simulink model "eval_ekf"  (R2026a)
settings: Solver=VariableStepAuto  StopTime=500
undefined symbols (not defined in the file): ekf_param, perturbed_plant_param, pf_param, r_param, random_seed, u_noise_param
libraries: lib_sensors x6, lib_plant x1
settings Model: SimulationMode=accelerator  Creator=alessandro-nardin  LastModifiedBy=fiore
settings RTWCC: Toolchain=Microsoft Visual C++ 2022 v17.0 | nmake (64-bit Windows)

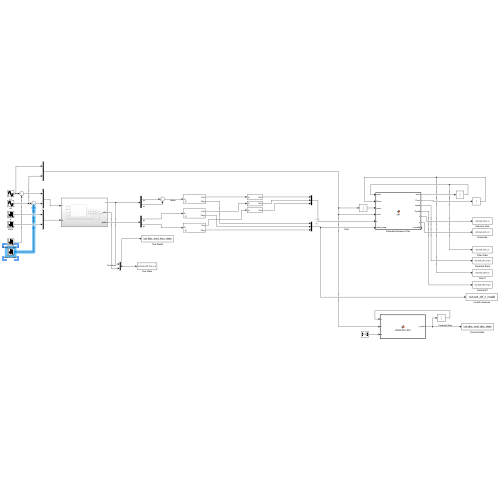
[thumbnail: Simulink's stored preview of the top-level diagram]
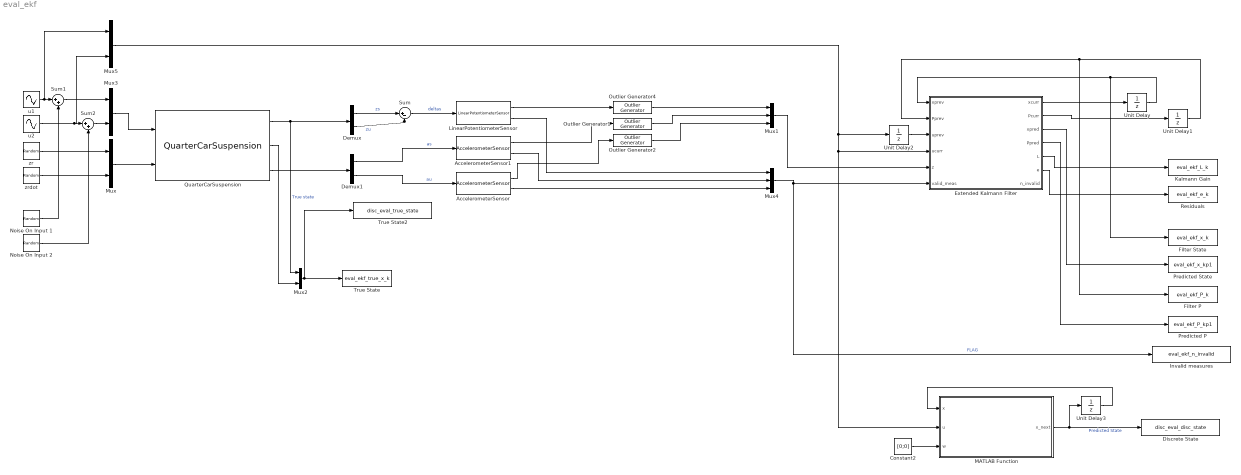
== system eval_ekf ==
  AccelerometerSensor : lib_sensors/AccelerometerSensor  out_sample_t=ekf_param.sample_t
  AccelerometerSensor1 : lib_sensors/AccelerometerSensor  out_sample_t=ekf_param.sample_t
  Constant2 : Constant  Value=[0;0]
  Demux : Demux  Outputs=2
  Demux1 : Demux  Outputs=2
  Discrete State : ToWorkspace  VariableName=disc_eval_disc_state  SaveFormat=Timeseries  SampleTime=ekf_param.sample_t
  Extended Kalmann Filter : MATLAB Function  TreatAsAtomicUnit=on
  Filter P : ToWorkspace  VariableName=eval_ekf_P_k  SaveFormat=Timeseries  SampleTime=1/ekf_param.freq
  Filter State : ToWorkspace  VariableName=eval_ekf_x_k  SaveFormat=Timeseries  SampleTime=1/ekf_param.freq
  Invalid measures : ToWorkspace  VariableName=eval_ekf_n_invalid  SaveFormat=Timeseries  SampleTime=ekf_param.sample_t
  Kalmann Gain : ToWorkspace  VariableName=eval_ekf_L_k  SaveFormat=Timeseries  SampleTime=pf_param.sample_t
  LinearPotentiometerSensor : lib_sensors/LinearPotentiometerSensor  out_sample_t=ekf_param.sample_t
  MATLAB Function : MATLAB Function  TreatAsAtomicUnit=on
  Mux{,2..3,5} (4 alike) : Mux  Inputs=2
  Mux1 : Mux  Inputs=3
  Mux4 : Mux  Inputs=3
  Noise On Input 1 : RandomNumber  Variance=u_noise_param.u1_var  Seed=random_seed+10  SampleTime=0
  Noise On Input 2 : RandomNumber  Variance=u_noise_param.u2_var  Seed=random_seed+10  SampleTime=0
  Outlier Generator1 : lib_sensors/Outlier Generator  outlier_probability=0.002  outlier_amplitude=5  sample_time=acc_param.sample_t
      settings: SourceProductName=Lib Sensors
  Outlier Generator2 : lib_sensors/Outlier Generator  outlier_probability=0.002  outlier_amplitude=5  sample_time=acc_param.sample_t
      settings: SourceProductName=Lib Sensors
  Outlier Generator4 : lib_sensors/Outlier Generator  outlier_probability=0.002  outlier_amplitude=5  sample_time=lpot_param.sample_t
      settings: SourceProductName=Lib Sensors
  Predicted P : ToWorkspace  VariableName=eval_ekf_P_kp1  SaveFormat=Timeseries  SampleTime=1/ekf_param.freq
  Predicted State : ToWorkspace  VariableName=eval_ekf_x_kp1  SaveFormat=Timeseries  SampleTime=1/ekf_param.freq
  QuarterCarSuspension : lib_plant/QuarterCarSuspension  SystemSampleTime=-1  VariantActivationTime=update diagram  EmptyChoice=off  PassThrough=off  PassThroughVariantControl=(default)  EmptyChoiceVariantControl=(default)  AllowFlexibleInterface=on  Latency=0  AutoFrameSizeCalculation=off
      settings: SourceProductName=Lib Plant
  Residuals : ToWorkspace  VariableName=eval_ekf_e_k  SaveFormat=Timeseries  SampleTime=-1
  Sum : Sum  Inputs=|+-
  Sum1 : Sum  Inputs=|++
  Sum2 : Sum  Inputs=|++
  True State : ToWorkspace  VariableName=eval_ekf_true_x_k  SaveFormat=Timeseries  SampleTime=1/ekf_param.freq
  True State2 : ToWorkspace  VariableName=disc_eval_true_state  SaveFormat=Timeseries  SampleTime=ekf_param.sample_t
  Unit Delay : UnitDelay  InitialCondition=ekf_param.x_init  SampleTime=ekf_param.sample_t
  Unit Delay1 : UnitDelay  InitialCondition=ekf_param.P_init  SampleTime=ekf_param.sample_t
  Unit Delay2 : UnitDelay  InitialCondition=[ 0; 0]  SampleTime=ekf_param.sample_t
  Unit Delay3 : UnitDelay  InitialCondition=[1;0;0;0]  SampleTime=ekf_param.sample_t
  u1 : Sin  Amplitude=943  Frequency=0.5  Phase=0.2  SampleTime=0
  u2 : Sin  Amplitude=2000  Phase=1  SampleTime=0
  zr : RandomNumber  Variance=r_param.rz_var  Seed=random_seed+6  SampleTime=0
  zrdot : RandomNumber  Variance=r_param.rzdot_var  Seed=random_seed+7  SampleTime=0
  wires:
  Demux/1 -> Sum/1  "zs"
  Demux/2 -> Sum/2  "zu"
  Sum/1 -> LinearPotentiometerSensor/1  "deltas"
  Demux1/2 -> AccelerometerSensor/1  "au"
  QuarterCarSuspension/3 -> Demux1/1
  Demux1/1 -> AccelerometerSensor1/1  "as"
  Mux/1 -> QuarterCarSuspension/2
  Extended Kalmann Filter/2(Pcurr) -> Unit Delay1/1
  Unit Delay1/1 -> Extended Kalmann Filter/2(Pprev), Filter P/1
  Unit Delay2/1 -> Extended Kalmann Filter/3(uprev)
  AccelerometerSensor1/1 -> Outlier Generator1/1
  Mux1/1 -> Extended Kalmann Filter/5(z)
  zr/1 -> Mux/1
  zrdot/1 -> Mux/2
  Unit Delay/1 -> Extended Kalmann Filter/1(xprev), Filter State/1
  Extended Kalmann Filter/1(xcurr) -> Unit Delay/1
  AccelerometerSensor/1 -> Outlier Generator2/1
  Mux4/1 -> Invalid measures/1, Extended Kalmann Filter/6(valid_meas)  "FLAG"
  LinearPotentiometerSensor/2 -> Mux4/1
  AccelerometerSensor1/2 -> Mux4/2
  AccelerometerSensor/2 -> Mux4/3
  LinearPotentiometerSensor/1 -> Outlier Generator4/1
  QuarterCarSuspension/2 -> Mux2/2
  Extended Kalmann Filter/3(xpred) -> Predicted State/1
  Extended Kalmann Filter/4(Ppred) -> Predicted P/1
  Extended Kalmann Filter/5(L) -> Kalmann Gain/1
  Extended Kalmann Filter/6(e) -> Residuals/1
  MATLAB Function/1(x_next) -> Discrete State/1, Unit Delay3/1  "Predicted State"
  Unit Delay3/1 -> MATLAB Function/1(x)
  Constant2/1 -> MATLAB Function/3(w)
  QuarterCarSuspension/1 -> Mux2/1, Demux/1  "True state"
  Mux2/1 -> True State2/1, True State/1
  Mux3/1 -> QuarterCarSuspension/1
  Sum1/1 -> Mux3/1
  u1/1 -> Mux5/1, Sum1/1
  Sum2/1 -> Mux3/2
  Noise On Input 2/1 -> Sum2/2
  Noise On Input 1/1 -> Sum1/2
  Mux5/1 -> MATLAB Function/2(u), Extended Kalmann Filter/4(ucurr), Unit Delay2/1
  u2/1 -> Mux5/2, Sum2/1
  Outlier Generator4/1 -> Mux1/1
  Outlier Generator1/1 -> Mux1/2
  Outlier Generator2/1 -> Mux1/3

== matlab function eval_ekf/MATLAB Function ==
  settings: updateMethod=DISCRETE  sampleTime=ekf_param.sample_t
  data: x input; u input; x_next output size=[ 4 1 ]; w input; perturbed_plant_param parameter; ekf_param parameter
function x_next = suspension_dics( x, u, w, perturbed_plant_param, ekf_param)
x_next = suspension_f_dics_euler( x, u, w, perturbed_plant_param, ekf_param.sample_t);

== matlab function eval_ekf/Extended Kalmann Filter ==
  settings: updateMethod=DISCRETE  sampleTime=ekf_param.sample_t
  data: xprev input; Pprev input; uprev input; ucurr input; z input; xcurr output size=[ 4 1 ]; Pcurr output; xpred output; Ppred output; perturbed_plant_param parameter; ekf_param parameter; L output; valid_meas input; e output; n_invalid output
function [ xcurr, Pcurr, xpred, Ppred, L, e, n_invalid ] = ekf( xprev, Pprev, uprev, ucurr, z, perturbed_plant_param, ekf_param, valid_meas)
[xcurr, Pcurr, xpred, Ppred, L, e, n_invalid] = ekf_step( xprev, Pprev, uprev, ucurr, z, perturbed_plant_param, ekf_param, valid_meas);
